simulink model "ball_balancing_platform"  (R2023b)
settings: Solver=VariableStepAuto  StartTime=0.0  StopTime=inf  RelTol=1e-3
values from neighbouring files (symbols this model uses):
  A = [0  1; 0  0]    [1-dof.mat]    (also in 2-dof.mat = [0 0 0 0 1 0 0 0 0 0 0 0 ... (16 elements, 4x4)]; ball_balancing_platform.mat = [0 0 0 0 0 0 0 0 0 0 0 0 ... (64 elements, 8x8)])
  B = [0 -0.1692]    [1-dof.mat]    (also in 2-dof.mat = [0  0; -0.253868468945  0; 0  0; 0  0.253868468945]; ball_balancing_platform.mat = [0 0 0 0 0 0 1 0 0 0 0 0 ... (16 elements, 8x2)])
  C = [1 0]    [1-dof.mat]    (also in 2-dof.mat = [1  0  0  0; 0  0  1  0]; ball_balancing_platform.mat = [1 0 0 0 0 1 0 0 0 0 1 0 ... (32 elements, 4x8)])
  D = 0    [1-dof.mat]    (also in 2-dof.mat = [0  0; 0  0]; ball_balancing_platform.mat = [0  0; 0  0; 0  0; 0  0])
libraries: robotlib x4, mpclib x1, aerolibanimutils x1
settings Model: Creator=farhan  LastModifiedBy=farhan

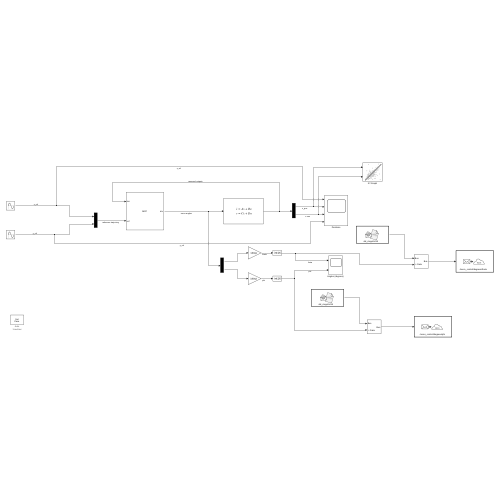
[thumbnail: Simulink's stored preview of the top-level diagram]
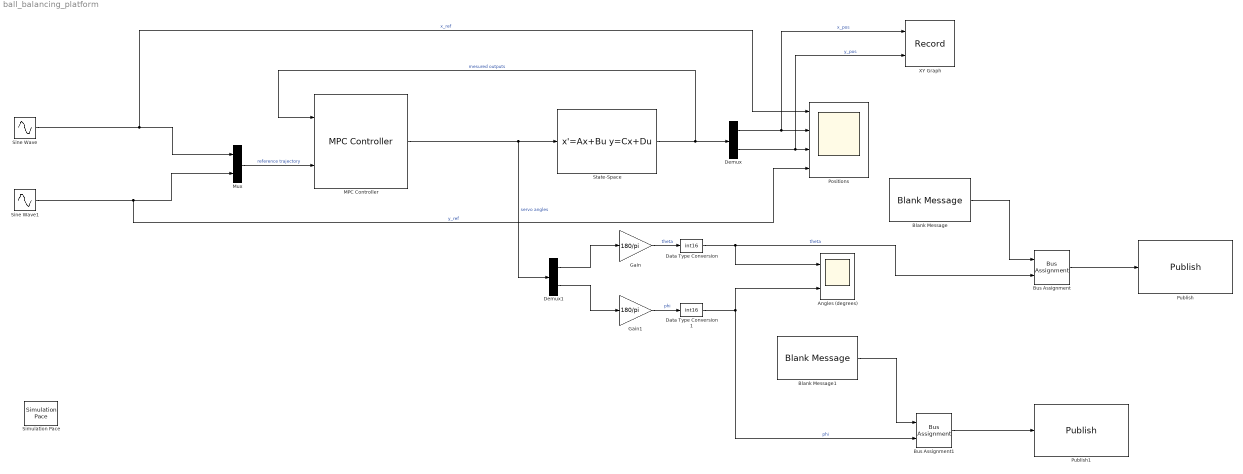
== system ball_balancing_platform ==
  Angles (degrees) : Scope  NumInputPorts=2
  Blank Message : robotlib/Blank Message  messageClass=Message  entityType=std_msgs/Int16  messageType=std_msgs/Int16  SampleTime=inf  legacyBusStruct=off
  Blank Message1 : robotlib/Blank Message  messageClass=Message  entityType=std_msgs/Int16  messageType=std_msgs/Int16  SampleTime=inf  legacyBusStruct=off
  Bus Assignment : BusAssignment  AssignedSignals=Data
  Bus Assignment1 : BusAssignment  AssignedSignals=Data
  Data Type Conversion : DataTypeConversion  OutDataTypeStr=int16  SaturateOnIntegerOverflow=off  RndMeth=Floor
  Data Type Conversion1 : DataTypeConversion  OutDataTypeStr=int16  SaturateOnIntegerOverflow=off  RndMeth=Floor
  Demux : Demux  Outputs=2
  Demux1 : Demux  Outputs=2
  Gain : Gain  Gain=180/pi
  Gain1 : Gain  Gain=180/pi
  MPC Controller : mpclib/MPC Controller  SCDEnableBlockLinearizationSpecification=on  mpcobj=mpc1  is_multiple=0  enable_value=0  return_u0=off  updateMPCinCallerWorkspace=on  md_inport=off  mv_inport=off  uref_inport=off  return_cost=off  return_mvseq=off  return_qpstatus=off  return_xseq=off  return_state=off  return_ovseq=off  state_inport=off  umin_inport=off  umax_inport=off  ymin_inport=off  ymax_inport=off  cc_inport=off  ywt_inport=off  uwt_inport=off  duwt_inport=off  rhoeps_inport=off  pm_inport=off  MaximumP=10  HorizonChoice=FixedHorizon  n_ts=0.1  n_p=6  n_mv=2  n_md=0  n_ud=0  n_mo=2  n_uo=0  BlockDataType=double  SampleTimeInherited=off  switch_inport=off
  Mux : Mux  Inputs=2
  Positions : Scope  NumInputPorts=4
  Publish : robotlib/Publish  topicSource=Specify your own  topic=/servo_control/degrees/theta  messageType=std_msgs/Int16  legacyBusStruct=off  messageQueueLength=1
  Publish1 : robotlib/Publish  topicSource=Specify your own  topic=/servo_control/degrees/phi  messageType=std_msgs/Int16  legacyBusStruct=off  messageQueueLength=1
  Simulation Pace : aerolibanimutils/Simulation Pace  SimulationPace=1  SleepMode=Auto  OutputPaceError=off  SampleTime=1/30
  Sine Wave : Sin  Amplitude=0.15  Frequency=0.5  SampleTime=0
  Sine Wave1 : Sin  Amplitude=-0.15  Frequency=0.5  Phase=pi/2  SampleTime=0
  State-Space : StateSpace  A=A  B=B  C=C  D=D  InitialCondition=[0; 0; 0; 0]
  XY Graph : Record  FileSettingsInternal="{\"entries\":[{\"content\":{\"excelSettings\":{\"content\":{},\"type\":\"Streamout.ExcelSettings\"}},\"type\":\"Streamout.FileSettingStorage\",\"uuid\":\"\"}],\"packageUris\":[\"http:\\/\\/schema.mathworks.com\\/mf0\\/streamout_blocks\\/R2020a\"],\"version\":\"1.0\"}"  Layout=[1 1]  SignalsInternal="{\"entries\":[{\"content\":{\"signals\":[{\"content\":{\"blockPath\":[],\"dimensions\":[1],\"domain\":\"\",\"lineColor\":\"#a2142f\",\"plots\":[1],\"port\":1,\"signalID\":17,\"signalName\":\"x_pos\"},\"type\":\"RecordBlkView.Signal\",\"uuid\":\"\"},{\"content\":{\"blockPath\":[],\"dimensions\":[1],\"domain\":\"\",\"lineColor\":\"#139fff\",\"plots\":[1],\"port\":2,\"signalID\":20,\"signalName\":\"y_pos\"},\"type\":\"RecordBlkView.Signal\",\"uuid\":\"\"}]},\"type\":\"RecordBlkView.InputSignals\",\"uuid\":\"\"}],\"packageUris\":[\"http:\\/\\/schema.mathworks.com\\/mf0\\/streamout_blocks\\/R2020a\"],\"version\":\"1.0\"}"  VisualizationBindings="{\"xyplotplugin\":{\"info\":[{\"series\":[{\"bindingParametersList\":[{\"parameter\":\"X-Axis\",\"signalID\":17,\"signalName\":\"x_pos\"},{\"parameter\":\"Y-Axis\",\"signalID\":20,\"signalName\":\"y_pos\"}],\"seriesID\":60889}],\"subplotID\":1}]}}"  CompatibilityTag=XY
  wires:
  MPC Controller/1 -> Demux1/1, State-Space/1  "servo angles"
  State-Space/1 -> Demux/1, MPC Controller/1  "mesured outputs"
  Mux/1 -> MPC Controller/2  "reference trajectory"
  Sine Wave/1 -> Positions/1, Mux/1  "x_ref"
  Sine Wave1/1 -> Mux/2, Positions/4  "y_ref"
  Demux/1 -> XY Graph/1, Positions/2  "x_pos"
  Demux/2 -> XY Graph/2, Positions/3  "y_pos"
  Demux1/1 -> Gain/1
  Demux1/2 -> Gain1/1
  Gain/1 -> Data Type Conversion/1  "theta"
  Gain1/1 -> Data Type Conversion1/1  "phi"
  Blank Message/1 -> Bus Assignment/1
  Bus Assignment/1 -> Publish/1
  Blank Message1/1 -> Bus Assignment1/1
  Bus Assignment1/1 -> Publish1/1
  Data Type Conversion/1 -> Angles (degrees)/1, Bus Assignment/2  "theta"
  Data Type Conversion1/1 -> Bus Assignment1/2, Angles (degrees)/2  "phi"
